simulink model "VER_PC_PARQUE_halow_UDP"  (R2022b)
settings: Solver=FixedStepDiscrete  StartTime=0.0  StopTime=inf  RelTol=1e-3
libraries: sldrtlib x4, dspnetwork x3, audiosources x1, audiofeatures x1, deeplib x1, simulink x1
settings Model: Creator=The MathWorks, Inc.  LastModifiedBy=Pacorajo
settings SolverCC: AlgebraicLoopSolver=TrustRegion  AutoInsertRateTranBlk=on  MaxZcPerStep=1
settings DataIOCC: LimitDataPoints=on  SaveOutput=off  SignalLogging=off  SaveTime=off
settings OptimizationCC: ReuseModelBlockBuffer=on  LifeSpan=inf  SimCompilerOptimization=on
settings DebuggingCC: AlgebraicLoopMsg=error  SingleTaskRateTransMsg=error  IntegerOverflowMsg=none  UnconnectedInputMsg=warning  UnconnectedOutputMsg=warning  UnconnectedLineMsg=warning  AllowSymbolicDim=off  SFUnexpectedBacktrackingDiag=warning  SFNoUnconditionalDefaultTransitionDiag=warning  SFExecutionAtInitializationDiag=none  IntegerSaturationMsg=none  ArithmeticOperatorsInVariantConditions=warning
settings ModelReferenceCC: EnableRefExpFcnMdlSchedulingChecks=on
settings SFSimCC: SimCtrlC=off  SimUseLocalCustomCode=off  CustomCodeUndefinedFunction=UseInterfaceOnly  SimTargetLang=C++
settings RTWCC: RTWUseLocalCustomCode=off  DLArmComputeVersion=19.05
settings CodeAppCC: StateflowObjectComments=on
settings GRTTargetCC: TargetLangStandard=C89/C90 (ANSI)
settings ConfigComp: CovMetricSettings=dw  CovSaveCumulativeToWorkspaceVar=on  CovSaveSingleToWorkspaceVar=on  CovExternalEMLEnable=off  CovSFcnEnable=off

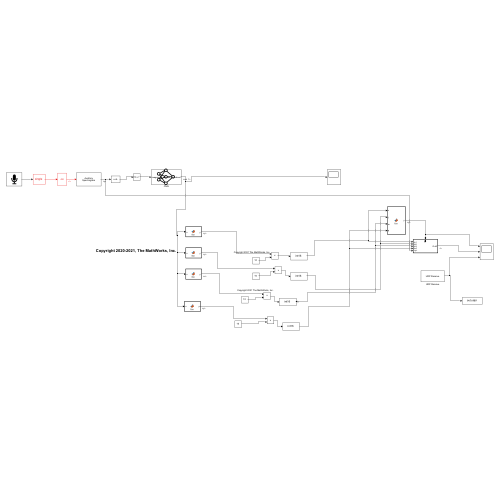
[thumbnail: Simulink's stored preview of the top-level diagram]
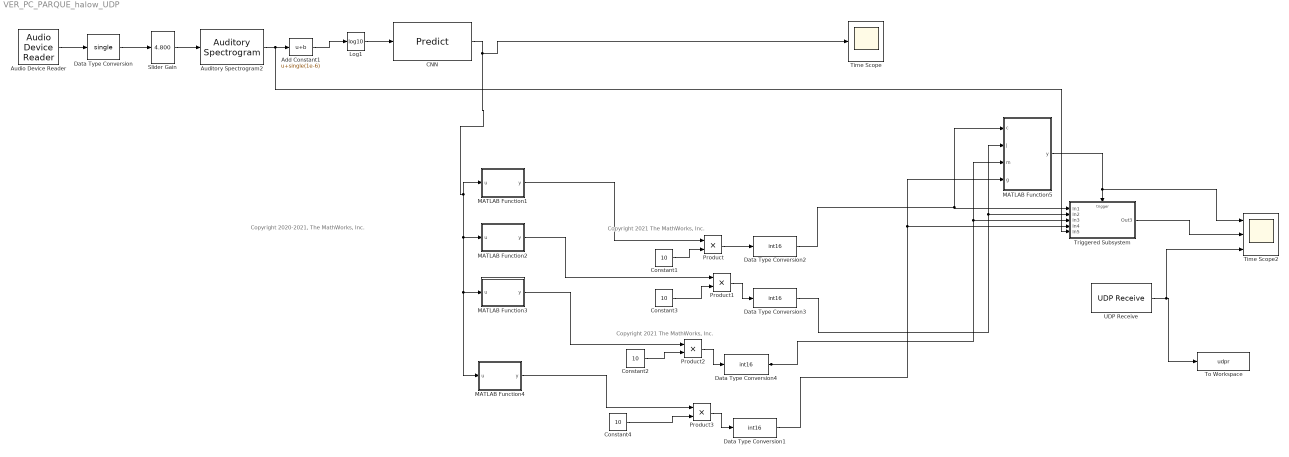
== system VER_PC_PARQUE_halow_UDP ==
  note: Copyright 2020-2021, The MathWorks, Inc.
  note: Copyright 2021 The MathWorks, Inc.
  note: Copyright 2021 The MathWorks, Inc.
  Add Constant1 : Bias  Bias=single(1e-6)  SaturateOnIntegerOverflow=off
  Audio Device Reader : audiosources/Audio Device Reader  Driver=DirectSound  Device=Default  SampleRate=16000  NumChannels=1  SamplesPerFrame=1600  BitDepth=16-bit integer  NumBuffers=10  DefaultInputChannelMapping=on  InputChannelMapping=1:2  OutputNumOverrunSamples=off  OutputDataType=double  DriverIdx=1  DeviceWarnFlag=''
  Auditory Spectrogram2 : audiofeatures/Auditory Spectrogram  FrequencyScale=bark  AutoNumBands=off  NumBands=50  AutoFrequencyRange=on  FrequencyRange=[0, 22050]  FilterBankDesignDomain=linear  FilterBankNormalization=bandwidth  OutputFrequencyVector=off  WindowParameter="hann(round(0.025*16e3),\"periodic\")"  WindowNormalization=off  OverlapLength=round(0.01*16e3)  AutoFFTLength=off  FFTLength=512  SpectrumType=power  NumHops=98  NumHopsOverlap=88  InheritSampleRate=off  SampleRate=16e3
  CNN : deeplib/Predict  Network=Network from MAT-file  NetworkFunction=squeezenet  NetworkFilePath=C:\demo\trained_parque.mat  MiniBatchSize=1  InputDataFormats={ '', '' }  Predictions=off  Activations={'softmax'}  ForceInterpretedSim=off  EnableDLNetwork=off
  Constant{1..4} (4 alike) : Constant  Value=10
  Data Type Conversion : DataTypeConversion  OutDataTypeStr=single  SaturateOnIntegerOverflow=off  RndMeth=Floor
  Data Type Conversion{1..4} (4 alike) : DataTypeConversion  OutDataTypeStr=int16  SaturateOnIntegerOverflow=off  RndMeth=Floor
  Log1 : Math  Operator=log10
  MATLAB Function1 : MATLAB Function  TreatAsAtomicUnit=on
  MATLAB Function2 : MATLAB Function  TreatAsAtomicUnit=on
  MATLAB Function3 : MATLAB Function  TreatAsAtomicUnit=on
  MATLAB Function4 : MATLAB Function  TreatAsAtomicUnit=on
  MATLAB Function5 : MATLAB Function  TreatAsAtomicUnit=on
  Product{,1..3} (4 alike) : Product
  Slider Gain : simulink/Math Operations/Slider Gain  gain=4.800  low=0  high=30
  Time Scope : Scope
  Time Scope2 : Scope  NumInputPorts=3
  To Workspace : ToWorkspace  VariableName=udpr  SaveFormat=Timeseries  SampleTime=-1
  Triggered Subsystem : Subsystem  TreatAsAtomicUnit=on
  UDP Receive : dspnetwork/UDP Receive  localURL='0.0.0.0'  localPort=25000  remoteURL='192.168.1.59'  remotePort=-1  recvBufferSize=8192*4  dims=4900  signalDatatype=single  isComplex=off  isVarSize=on  showBlockingTime=off  blockingTime=0  sampletime=1  blockPlatform=[]
      settings: LibrarySourceBlock=dspsrcs4/UDP Receive
  wires:
  Slider Gain/1 -> Auditory Spectrogram2/1
  Auditory Spectrogram2/1 -> Triggered Subsystem/5(In5), Add Constant1/1
  Add Constant1/1 -> Log1/1
  Log1/1 -> CNN/1
  MATLAB Function3/1(y) -> Product2/1
  MATLAB Function4/1(y) -> Product3/1
  Audio Device Reader/1 -> Data Type Conversion/1
  Data Type Conversion/1 -> Slider Gain/1
  Data Type Conversion4/1 -> Triggered Subsystem/3(In3), MATLAB Function5/3(m)
  Constant2/1 -> Product2/2
  Product2/1 -> Data Type Conversion4/1
  Data Type Conversion3/1 -> MATLAB Function5/2(j), Triggered Subsystem/2(In2)
  Product1/1 -> Data Type Conversion3/1
  Data Type Conversion2/1 -> MATLAB Function5/1(c), Triggered Subsystem/1(In1)
  Product/1 -> Data Type Conversion2/1
  Constant1/1 -> Product/2
  MATLAB Function1/1(y) -> Product/1
  MATLAB Function2/1(y) -> Product1/1
  Constant3/1 -> Product1/2
  Data Type Conversion1/1 -> MATLAB Function5/4(g), Triggered Subsystem/4(In4)
  Product3/1 -> Data Type Conversion1/1
  Constant4/1 -> Product3/2
  MATLAB Function5/1(y) -> Time Scope2/1, Triggered Subsystem/Trigger
  CNN/1 -> Time Scope/1, MATLAB Function4/1(u), MATLAB Function3/1(u), MATLAB Function2/1(u), MATLAB Function1/1(u)
  UDP Receive/1 -> Time Scope2/3, To Workspace/1
  Triggered Subsystem/1(Out3) -> Time Scope2/2

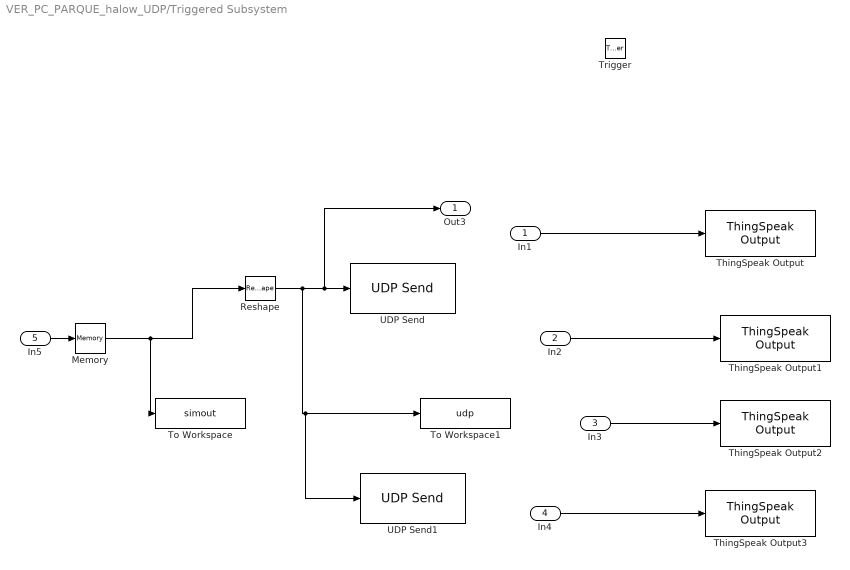
== system VER_PC_PARQUE_halow_UDP/Triggered Subsystem ==
  In1 : Inport
  In2 : Inport  Port=2
  In3 : Inport  Port=3
  In4 : Inport  Port=4
  In5 : Inport  Port=5
  Trigger : TriggerPort  VariantControl=(inherit)
  Memory : Memory  InheritSampleTime=on
  Reshape : Reshape  OutputDimensionality=Customize  OutputDimensions=[4900,1]
  ThingSpeak Output : sldrtlib/Internet of Things/ThingSpeak Output  DrvAddress=2363456  DrvOptions=[1 20 75 86 48 55 66 49 80 75 50 90 69 67 71 55 73 54 97 112 105 46 116 104 105 110 103 115 112 101 97 107 46 99 111 109 0 0 0 0 0 0 0 0 0 0 0 0 0 0 0 0 0 0 0 0 0 0 0 0 0 0 0 0 0 0 0 0 0 0 0 0 0 0 0 0 0 0 0 0 0 0 0 0 0 0 0 0 0 0 0 0 0 0 0 0 0 0 0 0 0 0 0 0 0 0 0 0 0 0 0 0 0 0 0 0 0 0 0 0 0 0 0 0 0 0 0 0 0 0 0 0 0 0 0 0 0 0 0 0 0 0 0 0 0 0 0 0 0 0 0 0 0 0 0 0 0 0 0 0 0 0 0 0 0 0 0 0 0 0 0 0 0 0 0 0 0 0 0 0 0 0 0 0 0 0 0 0 0 0 0 0 0 0 0 0 0 0 0 0 0 0 0 0 0 0 0 0 0 0 0 0 0 0 0 0 0 0 0 0 0 0 0 0 0 0 0 0 0 0 0 0 0 0 0 0 0 0 0 0 0 0 0 0 0 0 0 0 0 0 0 0 0 0 0 0]  SampleTime=-1  MaxMissedTicks=10  ShowMissedTicks=off  YieldWhenWaiting=off  ChannelFields=1  OptParam=0  InitialValue=[]  FinalValue=[]
  ThingSpeak Output1 : sldrtlib/Internet of Things/ThingSpeak Output  DrvAddress=2363456  DrvOptions=[1 20 75 86 48 55 66 49 80 75 50 90 69 67 71 55 73 54 97 112 105 46 116 104 105 110 103 115 112 101 97 107 46 99 111 109 0 0 0 0 0 0 0 0 0 0 0 0 0 0 0 0 0 0 0 0 0 0 0 0 0 0 0 0 0 0 0 0 0 0 0 0 0 0 0 0 0 0 0 0 0 0 0 0 0 0 0 0 0 0 0 0 0 0 0 0 0 0 0 0 0 0 0 0 0 0 0 0 0 0 0 0 0 0 0 0 0 0 0 0 0 0 0 0 0 0 0 0 0 0 0 0 0 0 0 0 0 0 0 0 0 0 0 0 0 0 0 0 0 0 0 0 0 0 0 0 0 0 0 0 0 0 0 0 0 0 0 0 0 0 0 0 0 0 0 0 0 0 0 0 0 0 0 0 0 0 0 0 0 0 0 0 0 0 0 0 0 0 0 0 0 0 0 0 0 0 0 0 0 0 0 0 0 0 0 0 0 0 0 0 0 0 0 0 0 0 0 0 0 0 0 0 0 0 0 0 0 0 0 0 0 0 0 0 0 0 0 0 0 0 0 0 0 0 0 0]  SampleTime=-1  MaxMissedTicks=10  ShowMissedTicks=off  YieldWhenWaiting=off  ChannelFields=2  OptParam=0  InitialValue=[]  FinalValue=[]
  ThingSpeak Output2 : sldrtlib/Internet of Things/ThingSpeak Output  DrvAddress=2363456  DrvOptions=[1 20 75 86 48 55 66 49 80 75 50 90 69 67 71 55 73 54 97 112 105 46 116 104 105 110 103 115 112 101 97 107 46 99 111 109 0 0 0 0 0 0 0 0 0 0 0 0 0 0 0 0 0 0 0 0 0 0 0 0 0 0 0 0 0 0 0 0 0 0 0 0 0 0 0 0 0 0 0 0 0 0 0 0 0 0 0 0 0 0 0 0 0 0 0 0 0 0 0 0 0 0 0 0 0 0 0 0 0 0 0 0 0 0 0 0 0 0 0 0 0 0 0 0 0 0 0 0 0 0 0 0 0 0 0 0 0 0 0 0 0 0 0 0 0 0 0 0 0 0 0 0 0 0 0 0 0 0 0 0 0 0 0 0 0 0 0 0 0 0 0 0 0 0 0 0 0 0 0 0 0 0 0 0 0 0 0 0 0 0 0 0 0 0 0 0 0 0 0 0 0 0 0 0 0 0 0 0 0 0 0 0 0 0 0 0 0 0 0 0 0 0 0 0 0 0 0 0 0 0 0 0 0 0 0 0 0 0 0 0 0 0 0 0 0 0 0 0 0 0 0 0 0 0 0 0]  SampleTime=-1  MaxMissedTicks=10  ShowMissedTicks=off  YieldWhenWaiting=off  ChannelFields=3  OptParam=0  InitialValue=[]  FinalValue=[]
  ThingSpeak Output3 : sldrtlib/Internet of Things/ThingSpeak Output  DrvAddress=2363456  DrvOptions=[1 20 75 86 48 55 66 49 80 75 50 90 69 67 71 55 73 54 97 112 105 46 116 104 105 110 103 115 112 101 97 107 46 99 111 109 0 0 0 0 0 0 0 0 0 0 0 0 0 0 0 0 0 0 0 0 0 0 0 0 0 0 0 0 0 0 0 0 0 0 0 0 0 0 0 0 0 0 0 0 0 0 0 0 0 0 0 0 0 0 0 0 0 0 0 0 0 0 0 0 0 0 0 0 0 0 0 0 0 0 0 0 0 0 0 0 0 0 0 0 0 0 0 0 0 0 0 0 0 0 0 0 0 0 0 0 0 0 0 0 0 0 0 0 0 0 0 0 0 0 0 0 0 0 0 0 0 0 0 0 0 0 0 0 0 0 0 0 0 0 0 0 0 0 0 0 0 0 0 0 0 0 0 0 0 0 0 0 0 0 0 0 0 0 0 0 0 0 0 0 0 0 0 0 0 0 0 0 0 0 0 0 0 0 0 0 0 0 0 0 0 0 0 0 0 0 0 0 0 0 0 0 0 0 0 0 0 0 0 0 0 0 0 0 0 0 0 0 0 0 0 0 0 0 0 0]  SampleTime=-1  MaxMissedTicks=10  ShowMissedTicks=off  YieldWhenWaiting=off  ChannelFields=4  OptParam=0  InitialValue=[]  FinalValue=[]
  To Workspace : ToWorkspace  VariableName=simout  SaveFormat=Timeseries  SampleTime=-1
  To Workspace1 : ToWorkspace  VariableName=udp  SaveFormat=Timeseries  SampleTime=-1
  UDP Send : dspnetwork/UDP Send  remoteURL='192.168.1.59'  remotePort=25000  localURL='0.0.0.0'  localPortSource=Automatically determine  localPort=-1  sendBufferSize=8192*4  sampletime=-1  blockPlatform=[]  separateLengthPort=0
      settings: LibrarySourceBlock=dspsnks4/UDP Send
  UDP Send1 : dspnetwork/UDP Send  remoteURL='192.168.1.59'  remotePort=25010  localURL='0.0.0.0'  localPortSource=Automatically determine  localPort=-1  sendBufferSize=8192*4  sampletime=-1  blockPlatform=[]  separateLengthPort=0
      settings: LibrarySourceBlock=dspsnks4/UDP Send
  Out3 : Outport
  wires:
  In1/1 -> ThingSpeak Output/1
  In3/1 -> ThingSpeak Output2/1
  In2/1 -> ThingSpeak Output1/1
  In4/1 -> ThingSpeak Output3/1
  Reshape/1 -> UDP Send1/1, To Workspace1/1, Out3/1, UDP Send/1
  Memory/1 -> Reshape/1, To Workspace/1
  In5/1 -> Memory/1

== matlab function VER_PC_PARQUE_halow_UDP/MATLAB Function2 ==
  data: u input; y output
function y = fcn(u)
y= u(:,1,3) 
end

== matlab function VER_PC_PARQUE_halow_UDP/MATLAB Function1 ==
  data: u input; y output
function y = fcn(u)
y= u(:,1,2) 
end

== matlab function VER_PC_PARQUE_halow_UDP/MATLAB Function3 ==
  data: u input; y output
function y = fcn(u)
y= u(:,1,4) 
end

== matlab function VER_PC_PARQUE_halow_UDP/MATLAB Function4 ==
  data: u input; y output
function y = fcn(u)
y= u(:,1,5) 
end

== matlab function VER_PC_PARQUE_halow_UDP/MATLAB Function5 ==
  data: c input; y output; j input; m input; g input
function y = fcn(c,j,m,g)
y=0;
if ((c > 5 || j > 5 || m > 5|| g > 5) & y==0)
    y=1;
    
else
    y=0;
    
end;
